simulink model "Full_model_M_function_spring_stiffness"  (R2018a)
settings: Solver=VariableStepAuto  StartTime=0.0  StopTime=10.0  FixedStep=0.00000001  RelTol=1e-3
values from neighbouring files (symbols this model uses):
  bs = 2000    [Full_model_M_function_spring_stiffness.mat]
  bse = 3000    [Full_model_M_function_spring_stiffness.mat]
  Kse = 8000    [Full_model_M_function_spring_stiffness.mat]
  Kt = 125000    [Full_model_M_function_spring_stiffness.mat]
  Ms = 250    [Full_model_M_function_spring_stiffness.mat]
  Mse = 90    [Full_model_M_function_spring_stiffness.mat]
  Mu = 40    [Full_model_M_function_spring_stiffness.mat]
  poly_coeffs = [-5674000000 1562000000 -148500000 6452000 -136500 3607 -2.036]    [Full_model_M_function_spring_stiffness.mat]
  x_data = [9.36492633169e-06 0.00052288405136 0.00126203754344 0.00219289677269 0.00306560277016 0.00370561433637 0.00457832033384 0.00562556753081 0.00667289623196 0.00766199019716 0.0087673906259 0.00987279105464 ... (153 elements, 153x1)]    [Full_model_M_function_spring_stiffness.mat]
  x_pivot = 0.1    [Full_model_M_function_spring_stiffness.mat]
  y_data = [0.353838795839 1.64664314562 3.64098353081 5.62651628015 7.61181614974 9.19982316566 11.1851230353 13.5674828788 16.3462040569 18.7283310207 21.110923744 23.4935164672 ... (153 elements, 153x1)]    [Full_model_M_function_spring_stiffness.mat]
  ypivot = 541.664    [Full_model_M_function_spring_stiffness.mat]
  Zr = 0.2    [Full_model_M_function_spring_stiffness.mat]
settings Model: Creator=Saurabh Suman  LastModifiedBy=Saurabh Suman

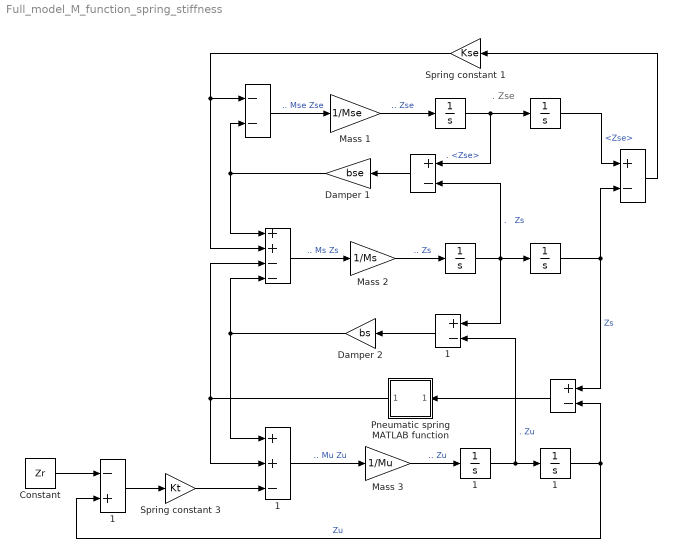
== system Full_model_M_function_spring_stiffness ==
  note: .
      | Zse
  " " : Integrator
  "  " : Sum  Inputs=+-
  "     " : Integrator
  "      " : Sum  Inputs=++--
  "       " : Sum  Inputs=--
  "        " : Sum  Inputs=+-
  "         " : Integrator
  "          " : Integrator
  "             " : Sum  Inputs=+-
  "             1" : Sum  Inputs=+-
  "          1" : Integrator
  "         1" : Integrator
  "       1" : Sum  Inputs=-+
  "      1" : Sum  Inputs=++-
  Constant : Constant  Value=Zr
  Damper 1 : Gain  Gain=bse
  Damper 2 : Gain  Gain=bs
  Mass 1 : Gain  Gain=1/Mse
  Mass 2 : Gain  Gain=1/Ms
  Mass 3 : Gain  Gain=1/Mu
  Pneumatic spring MATLAB function : Subsystem
  Spring constant 1 : Gain  Gain=Kse
  Spring constant 3 : Gain  Gain=Kt
  wires:
  "     "/1 -> "  "/1  "<Zse>"
  "       1"/1 -> Spring constant 3/1
  " "/1 -> "        "/1, "     "/1  ". <Zse>"
  Mass 1/1 -> " "/1  ".. Zse"
  Damper 1/1 -> "      "/1, "       "/2
  Damper 2/1 -> "      1"/1, "      "/4
  Spring constant 3/1 -> "      1"/3
  "          "/1 -> "             "/1, "  "/2  "Zs"
  "      1"/1 -> Mass 3/1  ".. Mu Zu"
  "       "/1 -> Mass 1/1  ".. Mse Zse"
  Mass 3/1 -> "         1"/1  ".. Zu"
  "             1"/1 -> Damper 2/1
  "  "/1 -> Spring constant 1/1
  "         1"/1 -> "          1"/1, "             1"/2  ". Zu"
  "          1"/1 -> "       1"/2, "             "/2  "Zu"
  Constant/1 -> "       1"/1
  Spring constant 1/1 -> "      "/2, "       "/1
  "      "/1 -> Mass 2/1  ".. Ms Zs"
  Mass 2/1 -> "         "/1  ".. Zs"
  "         "/1 -> "        "/2, "          "/1, "             1"/1  ".   Zs"
  "        "/1 -> Damper 1/1
  Pneumatic spring MATLAB function/1(Out1) -> "      1"/2, "      "/3
  "             "/1 -> Pneumatic spring MATLAB function/1(In1)

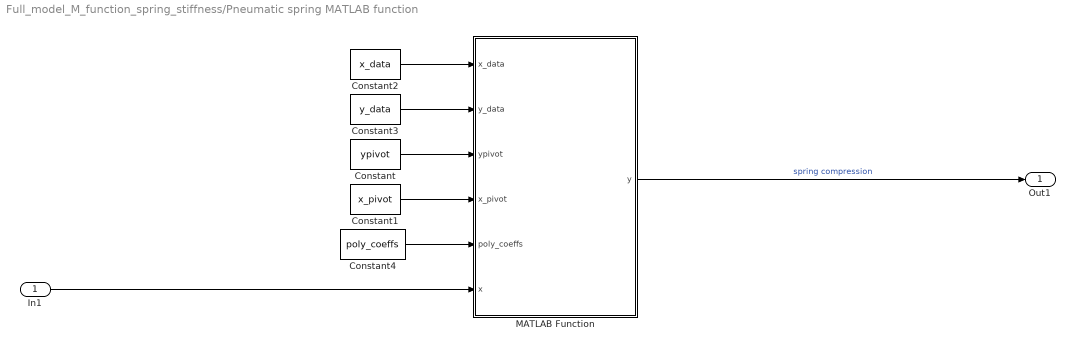
== system Full_model_M_function_spring_stiffness/Pneumatic spring MATLAB function ==
  In1 : Inport
  Constant : Constant  Value=ypivot  VectorParams1D=off
  Constant1 : Constant  Value=x_pivot  VectorParams1D=off
  Constant2 : Constant  Value=x_data  VectorParams1D=off
  Constant3 : Constant  Value=y_data  VectorParams1D=off
  Constant4 : Constant  Value=poly_coeffs  VectorParams1D=off
  MATLAB Function : MATLAB Function  TreatAsAtomicUnit=on
  Out1 : Outport
  wires:
  MATLAB Function/1(y) -> Out1/1  "spring compression"
  In1/1 -> MATLAB Function/6(x)
  Constant4/1 -> MATLAB Function/5(poly_coeffs)
  Constant1/1 -> MATLAB Function/4(x_pivot)
  Constant3/1 -> MATLAB Function/2(y_data)
  Constant2/1 -> MATLAB Function/1(x_data)
  Constant/1 -> MATLAB Function/3(ypivot)

== matlab function Full_model_M_function_spring_stiffness/Pneumatic spring MATLAB function/MATLAB Function ==
  data: x_data input; y_data input; ypivot input; x_pivot input; poly_coeffs input; x input; y output
function y = poly_limited(x_data, y_data, ypivot, x_pivot, poly_coeffs, x)
% Polynomial region
ypoly = polyval(poly_coeffs, x);
y1 = interp1(x_data, y_data, x_pivot);
y2 = interp1(x_data, y_data, x_pivot-0.01);
dfdx = (y2 -y1) / 0.01;

if x < 0
    y = 0;
elseif x <= x_pivot
    y = ypoly;
else
    y = ypivot + dfdx * (x - x_pivot);  % Linear extrapolation
end
